simulink subsystem "Simulatorev2slx"  (R2023a)
settings: Solver=VariableStepAuto  StartTime=0.0  StopTime=10.0  RelTol=1e-3
model mask{rho=971, rho_air=971, c_p=4179, c_p_air=4179, pi=3.14151, L_F=40.5, D_F=0.4, h_F=1.5, D_S1=0.1, L_S1=5, h_S1=1.5, D_S2=0.02, L_S2=50, h_S2=1.5, D_S3=0.1, L_S3=5, h_S3=1.5, D_R=0.4, L_R=40, h_R=1.5, V_b=300, A_b=500, h_b=1.5, T_F_0=273, T_S1_0=273, T_S2_0=273, T_S3_0=273, T_b_0=273, T_R_0=273}
  mask prompts: rho "rho water [kg/m^3]"; rho_air "rho air [kg/m^3]"; c_p "c_p water [J/kgK]"; c_p_air "c_p air [J/kgK]"; L_F "Length of F [m]"; D_F "Diameter of F [m]"; h_F "h_F [W/m^2K]"; D_S1 "Diameter of S1 [m]"; L_S1 "Length of S1"; D_S2 "Diameter of S2"; L_S2 "Length of S2"; D_S3 "Diameter of S3"; L_S3 "Length of S3"; D_R "Diameter of R"; L_R "Length of R"; V_b "V_building"; A_b "A_building_hull"; h_b "h_building"
undefined symbols (not defined in the file): C_b, C_F, C_R, C_S1, C_S2, C_S3, k_b, k_F, k_R, k_S1, k_S2, k_S3
settings Model: Creator=alex  LastModifiedBy=alex
settings OptimizationCC: ReuseModelBlockBuffer=off

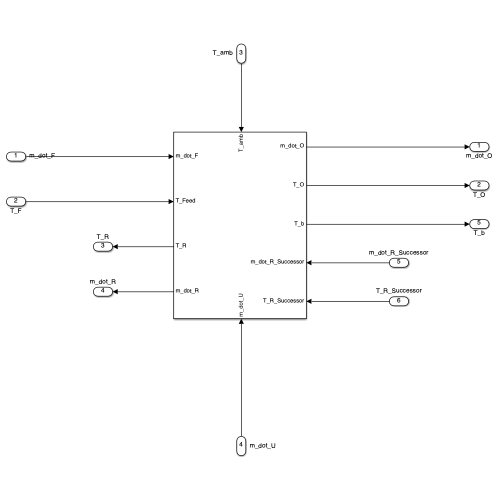
[thumbnail: Simulink's stored preview of the top-level diagram]
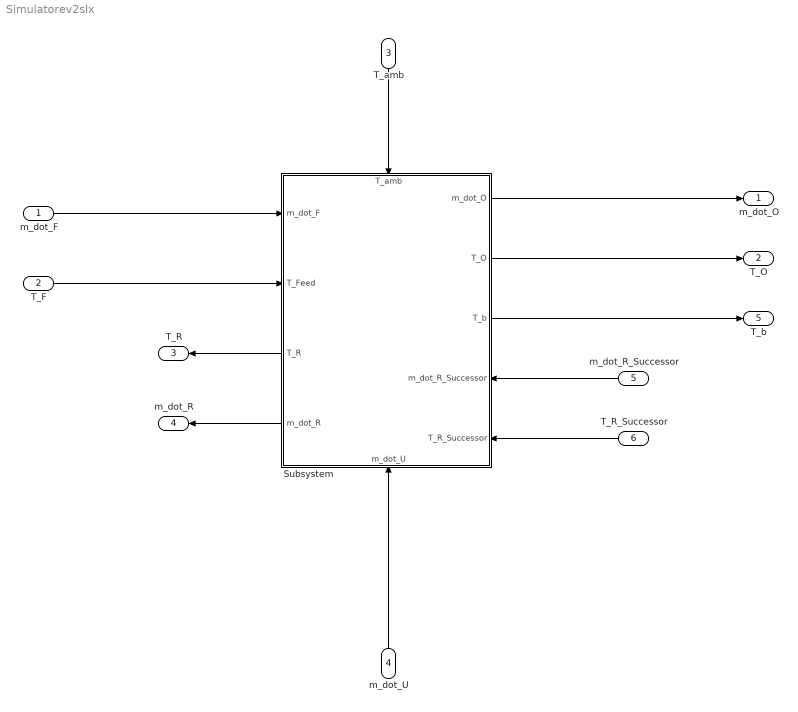
== system Simulatorev2slx ==
  m_dot_F : Inport
  T_F : Inport  Port=2
  T_amb : Inport  Port=3
  m_dot_U : Inport  Port=4
  m_dot_R_Successor : Inport  Port=5
  T_R_Successor : Inport  Port=6
  Subsystem : Subsystem
      settings: PortSchema="{\"entries\":[{\"content\":{\"sides\":[{\"content\":{\"connectorIds\":[\"In1\",\"In2\",\"Out4\",\"Out5\"]},\"type\":\"ConnectorPlacement.EquallySpacedRectSide\",\"uuid\":\"02066a73-e12c-4efb-ac1f-3567aea7908b\"},{\"content\":{\"connectorIds\":[\"Out1\",\"Out2\",\"Out3\",\"In5\",\"In6\"],\"side\":\"RIGHT\"},\"type\":\"ConnectorPlacement.EquallySpacedRectSide\",\"uuid\":\"ccd81727-46b8-449c-bb2a-a5652a5d9084\"},{\"content\":{\"connectorIds\":[\"In3\"],\"side\":\"TOP\"},\"type\":\"ConnectorPlacement.EquallySpacedRectSide\",\"uuid\":\"9b852ef9-fe85-43d4-afda-854933deff9c\"},{\"content\":{\"connectorIds\":[\"In4\"],\"side\":\"BOTTOM\"},\"type\":\"ConnectorPlacement.EquallySpacedRectSide\",\"uuid\":\"c5c6073a-07c2-439b-a52e-85716bb20a3c\"}]},\"type\":\"ConnectorPlacement.EquallySpacedConnector\",\"uuid\":\"28865625-48f4-4f1f-9e76-2e1450716591\"}],\"packageUris\":[\"http://schema.mathworks.com/mf0/Connector/R2020b\"],\"version\":\"1.0\"}"
  m_dot_O : Outport
  T_O : Outport  Port=2
  T_R : Outport  Port=3
  m_dot_R : Outport  Port=4
  T_b : Outport  Port=5
  wires:
  m_dot_F/1 -> Subsystem/1(m_dot_F)
  T_F/1 -> Subsystem/2(T_Feed)
  T_amb/1 -> Subsystem/3(T_amb)
  m_dot_U/1 -> Subsystem/4(m_dot_U)
  Subsystem/1(m_dot_O) -> m_dot_O/1
  Subsystem/2(T_O) -> T_O/1
  m_dot_R_Successor/1 -> Subsystem/5(m_dot_R_Successor)
  T_R_Successor/1 -> Subsystem/6(T_R_Successor)
  Subsystem/4(T_R) -> T_R/1
  Subsystem/5(m_dot_R) -> m_dot_R/1
  Subsystem/3(T_b) -> T_b/1

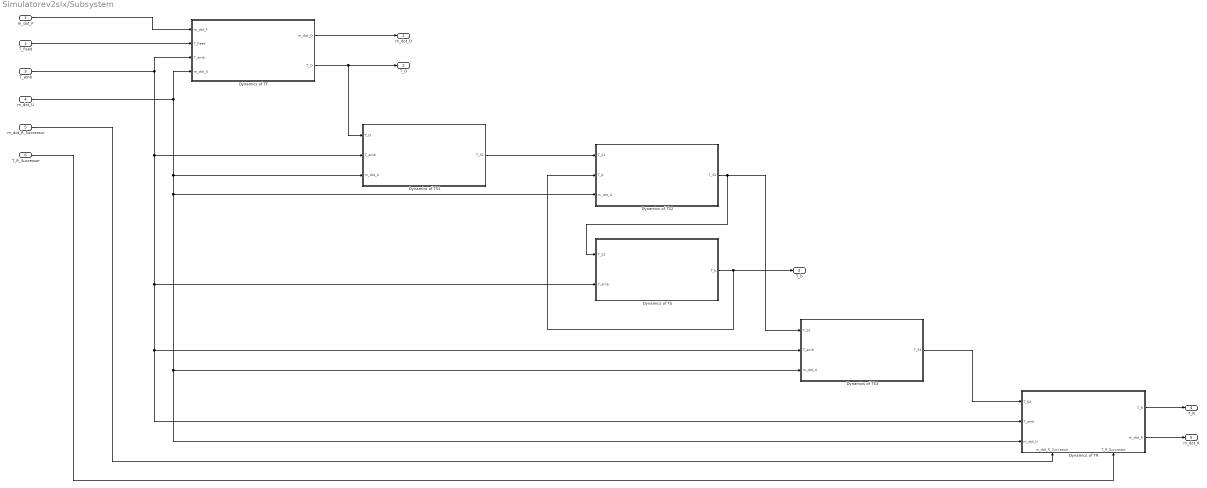
== system Simulatorev2slx/Subsystem ==
  m_dot_F : Inport
  T_Feed : Inport  Port=2
  T_amb : Inport  Port=3
  m_dot_U : Inport  Port=4
  m_dot_R_Successor : Inport  Port=5
  T_R_Successor : Inport  Port=6
  Dynamics of TF : Subsystem
  Dynamics of TR : Subsystem
      settings: PortSchema="{\"entries\":[{\"content\":{\"sides\":[{\"content\":{\"connectorIds\":[\"In1\",\"In2\",\"In3\"]},\"type\":\"ConnectorPlacement.EquallySpacedRectSide\",\"uuid\":\"1d5cfb0c-3444-494a-8f15-ea1ce9aa89e1\"},{\"content\":{\"connectorIds\":[\"Out1\",\"Out2\"],\"side\":\"RIGHT\"},\"type\":\"ConnectorPlacement.EquallySpacedRectSide\",\"uuid\":\"a241c28b-af63-4b6d-8a8e-9e454c2f304f\"},{\"content\":{\"side\":\"TOP\"},\"type\":\"ConnectorPlacement.EquallySpacedRectSide\",\"uuid\":\"7a4239f2-e3be-4ccc-ba79-85038cac89dd\"},{\"content\":{\"connectorIds\":[\"In4\",\"In5\"],\"side\":\"BOTTOM\"},\"type\":\"ConnectorPlacement.EquallySpacedRectSide\",\"uuid\":\"03da5dbc-12e1-4117-b594-812fe8cbcf6d\"}]},\"type\":\"ConnectorPlacement.EquallySpacedConnector\",\"uuid\":\"6bf2d3a5-b163-467e-ac11-ed480dce725b\"}],\"packageUris\":[\"http://schema.mathworks.com/mf0/Connector/R2020b\"],\"version\":\"1.0\"}"
  Dynamics of TS1 : Subsystem
  Dynamics of TS2 : Subsystem
  Dynamics of TS3 : Subsystem
  Dynamics of Tb : Subsystem
  m_dot_O : Outport
  T_O : Outport  Port=2
  T_b : Outport  Port=3
  T_R : Outport  Port=4
  m_dot_R : Outport  Port=5
  wires:
  m_dot_F/1 -> Dynamics of TF/1(m_dot_F)
  T_Feed/1 -> Dynamics of TF/2(T_Feed)
  T_amb/1 -> Dynamics of Tb/2(T_amb), Dynamics of TS3/2(T_amb), Dynamics of TR/2(T_amb), Dynamics of TS1/2(T_amb), Dynamics of TF/3(T_amb)
  m_dot_U/1 -> Dynamics of TR/3(m_dot_U), Dynamics of TS3/3(m_dot_U), Dynamics of TS2/3(m_dot_U), Dynamics of TS1/3(m_dot_U), Dynamics of TF/4(m_dot_U)
  Dynamics of TF/1(m_dot_O) -> m_dot_O/1
  Dynamics of TF/2(T_O) -> Dynamics of TS1/1(T_O), T_O/1
  Dynamics of TS1/1(T_S1) -> Dynamics of TS2/1(T_S1)
  Dynamics of TS2/1(T_S2) -> Dynamics of TS3/1(T_S2), Dynamics of Tb/1(T_S2)
  Dynamics of Tb/1(T_b) -> T_b/1, Dynamics of TS2/2(T_b)
  m_dot_R_Successor/1 -> Dynamics of TR/4(m_dot_R_Successor)
  T_R_Successor/1 -> Dynamics of TR/5(T_R_Successor)
  Dynamics of TS3/1(T_S3) -> Dynamics of TR/1(T_S3)
  Dynamics of TR/1(T_R) -> T_R/1
  Dynamics of TR/2(m_dot_R) -> m_dot_R/1

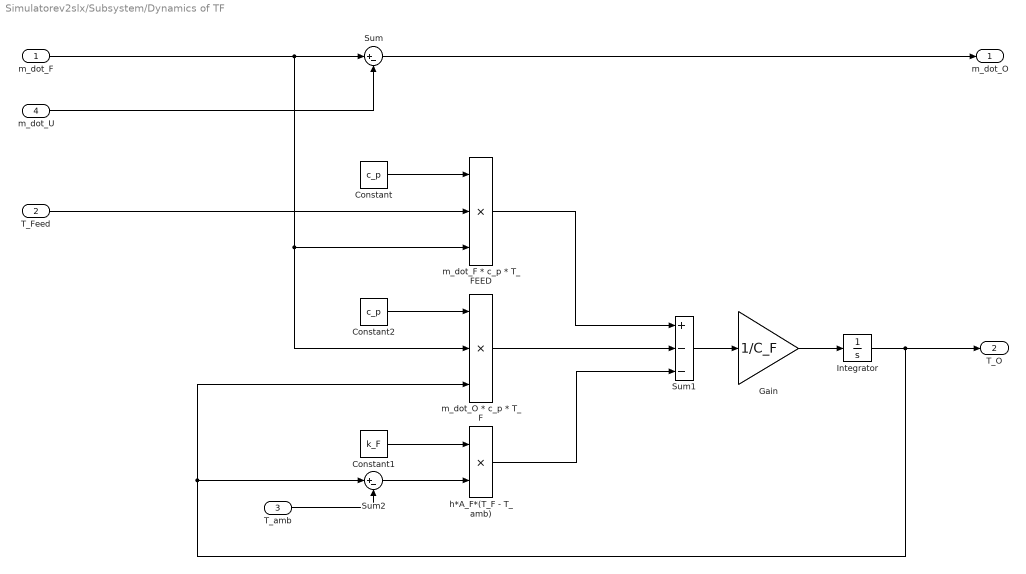
== system Simulatorev2slx/Subsystem/Dynamics of TF ==
  m_dot_F : Inport
  T_Feed : Inport  Port=2
  T_amb : Inport  Port=3
  m_dot_U : Inport  Port=4
  Constant : Constant  Value=c_p
  Constant1 : Constant  Value=k_F
  Constant2 : Constant  Value=c_p
  Gain : Gain  Gain=1/C_F
  Integrator : Integrator  InitialCondition=T_F_0
  Sum : Sum  Inputs=|+-
  Sum1 : Sum  Inputs=+--
  Sum2 : Sum  Inputs=|+-
  h*A_F*(T_F - T_amb) : Product
  m_dot_F * c_p * T_FEED : Product  Inputs=3
  m_dot_O * c_p * T_F : Product  Inputs=3
  m_dot_O : Outport
  T_O : Outport  Port=2
  wires:
  Constant2/1 -> m_dot_O * c_p * T_F/1
  m_dot_O * c_p * T_F/1 -> Sum1/2
  T_amb/1 -> Sum2/2
  Integrator/1 -> T_O/1, m_dot_O * c_p * T_F/3, Sum2/1
  Constant1/1 -> h*A_F*(T_F - T_amb)/1
  h*A_F*(T_F - T_amb)/1 -> Sum1/3
  Sum2/1 -> h*A_F*(T_F - T_amb)/2
  m_dot_F * c_p * T_FEED/1 -> Sum1/1
  Constant/1 -> m_dot_F * c_p * T_FEED/1
  Sum1/1 -> Gain/1
  m_dot_F/1 -> m_dot_F * c_p * T_FEED/3, m_dot_O * c_p * T_F/2, Sum/1
  Gain/1 -> Integrator/1
  Sum/1 -> m_dot_O/1
  T_Feed/1 -> m_dot_F * c_p * T_FEED/2
  m_dot_U/1 -> Sum/2

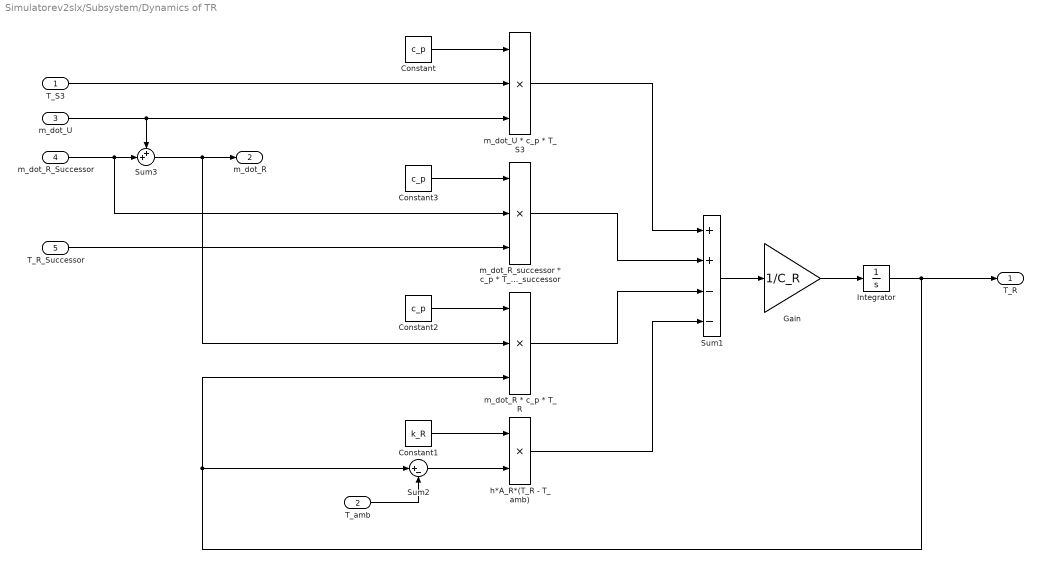
== system Simulatorev2slx/Subsystem/Dynamics of TR ==
  T_S3 : Inport
  T_amb : Inport  Port=2
  m_dot_U : Inport  Port=3
  m_dot_R_Successor : Inport  Port=4
  T_R_Successor : Inport  Port=5
  Constant : Constant  Value=c_p
  Constant1 : Constant  Value=k_R
  Constant2 : Constant  Value=c_p
  Constant3 : Constant  Value=c_p
  Gain : Gain  Gain=1/C_R
  Integrator : Integrator  InitialCondition=T_R_0
  Sum1 : Sum  Inputs=++--
  Sum2 : Sum  Inputs=|+-
  Sum3 : Sum  Inputs=++|
  h*A_R*(T_R - T_amb) : Product
  m_dot_R * c_p * T_R : Product  Inputs=3
  m_dot_R_successor * c_p * T_R_successor : Product  Inputs=3
  m_dot_U * c_p * T_S3 : Product  Inputs=3
  T_R : Outport
  m_dot_R : Outport  Port=2
  wires:
  Constant2/1 -> m_dot_R * c_p * T_R/1
  T_amb/1 -> Sum2/2
  Integrator/1 -> T_R/1, m_dot_R * c_p * T_R/3, Sum2/1
  Constant1/1 -> h*A_R*(T_R - T_amb)/1
  Sum2/1 -> h*A_R*(T_R - T_amb)/2
  Constant/1 -> m_dot_U * c_p * T_S3/1
  Sum1/1 -> Gain/1
  Gain/1 -> Integrator/1
  T_S3/1 -> m_dot_U * c_p * T_S3/2
  m_dot_U/1 -> m_dot_U * c_p * T_S3/3, Sum3/1
  Sum3/1 -> m_dot_R * c_p * T_R/2, m_dot_R/1
  m_dot_R_Successor/1 -> m_dot_R_successor * c_p * T_R_successor/2, Sum3/2
  Constant3/1 -> m_dot_R_successor * c_p * T_R_successor/1
  T_R_Successor/1 -> m_dot_R_successor * c_p * T_R_successor/3
  h*A_R*(T_R - T_amb)/1 -> Sum1/4
  m_dot_R * c_p * T_R/1 -> Sum1/3
  m_dot_R_successor * c_p * T_R_successor/1 -> Sum1/2
  m_dot_U * c_p * T_S3/1 -> Sum1/1

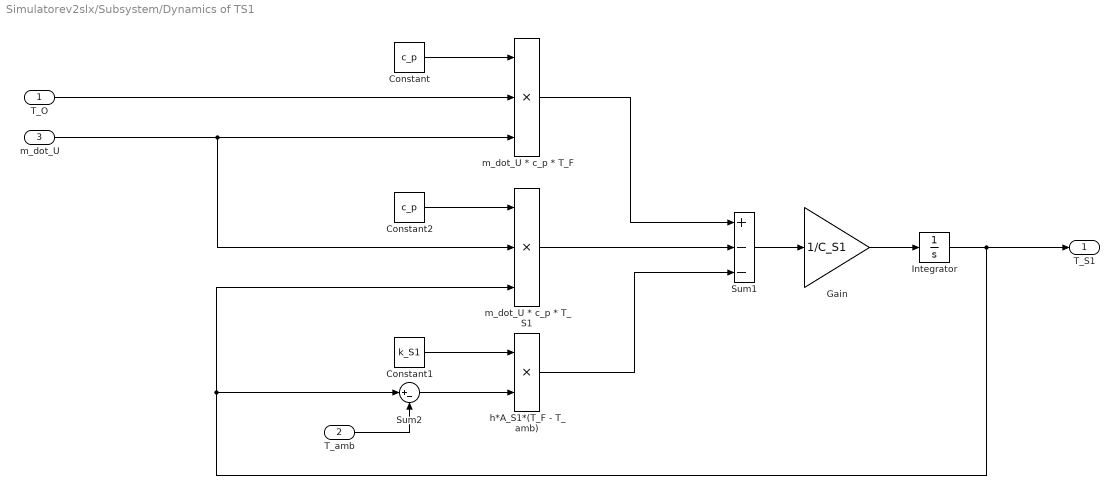
== system Simulatorev2slx/Subsystem/Dynamics of TS1 ==
  T_O : Inport
  T_amb : Inport  Port=2
  m_dot_U : Inport  Port=3
  Constant : Constant  Value=c_p
  Constant1 : Constant  Value=k_S1
  Constant2 : Constant  Value=c_p
  Gain : Gain  Gain=1/C_S1
  Integrator : Integrator  InitialCondition=T_S1_0
  Sum1 : Sum  Inputs=+--
  Sum2 : Sum  Inputs=|+-
  h*A_S1*(T_F - T_amb) : Product
  m_dot_U * c_p * T_F : Product  Inputs=3
  m_dot_U * c_p * T_S1 : Product  Inputs=3
  T_S1 : Outport
  wires:
  Constant2/1 -> m_dot_U * c_p * T_S1/1
  m_dot_U * c_p * T_S1/1 -> Sum1/2
  T_amb/1 -> Sum2/2
  Integrator/1 -> T_S1/1, m_dot_U * c_p * T_S1/3, Sum2/1
  Constant1/1 -> h*A_S1*(T_F - T_amb)/1
  h*A_S1*(T_F - T_amb)/1 -> Sum1/3
  Sum2/1 -> h*A_S1*(T_F - T_amb)/2
  m_dot_U * c_p * T_F/1 -> Sum1/1
  Constant/1 -> m_dot_U * c_p * T_F/1
  Sum1/1 -> Gain/1
  Gain/1 -> Integrator/1
  T_O/1 -> m_dot_U * c_p * T_F/2
  m_dot_U/1 -> m_dot_U * c_p * T_S1/2, m_dot_U * c_p * T_F/3

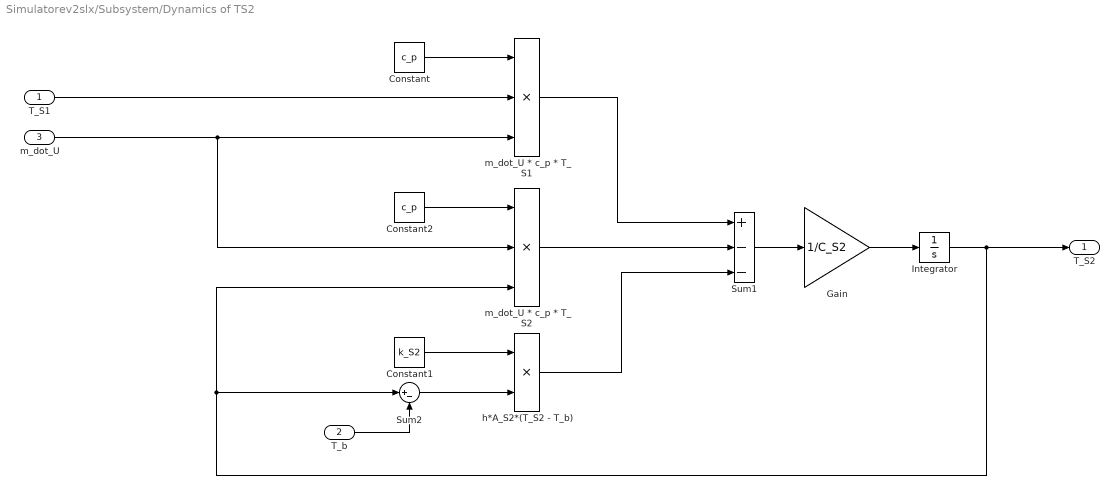
== system Simulatorev2slx/Subsystem/Dynamics of TS2 ==
  T_S1 : Inport
  T_b : Inport  Port=2
  m_dot_U : Inport  Port=3
  Constant : Constant  Value=c_p
  Constant1 : Constant  Value=k_S2
  Constant2 : Constant  Value=c_p
  Gain : Gain  Gain=1/C_S2
  Integrator : Integrator  InitialCondition=T_S2_0
  Sum1 : Sum  Inputs=+--
  Sum2 : Sum  Inputs=|+-
  h*A_S2*(T_S2 - T_b) : Product
  m_dot_U * c_p * T_S1 : Product  Inputs=3
  m_dot_U * c_p * T_S2 : Product  Inputs=3
  T_S2 : Outport
  wires:
  Constant2/1 -> m_dot_U * c_p * T_S2/1
  m_dot_U * c_p * T_S2/1 -> Sum1/2
  T_b/1 -> Sum2/2
  Integrator/1 -> T_S2/1, m_dot_U * c_p * T_S2/3, Sum2/1
  Constant1/1 -> h*A_S2*(T_S2 - T_b)/1
  h*A_S2*(T_S2 - T_b)/1 -> Sum1/3
  Sum2/1 -> h*A_S2*(T_S2 - T_b)/2
  m_dot_U * c_p * T_S1/1 -> Sum1/1
  Constant/1 -> m_dot_U * c_p * T_S1/1
  Sum1/1 -> Gain/1
  Gain/1 -> Integrator/1
  T_S1/1 -> m_dot_U * c_p * T_S1/2
  m_dot_U/1 -> m_dot_U * c_p * T_S2/2, m_dot_U * c_p * T_S1/3

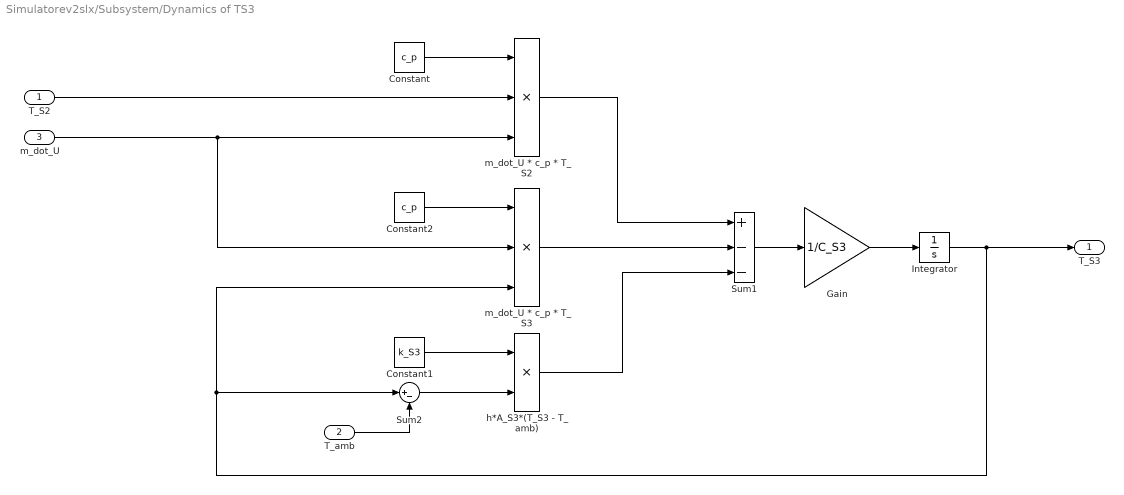
== system Simulatorev2slx/Subsystem/Dynamics of TS3 ==
  T_S2 : Inport
  T_amb : Inport  Port=2
  m_dot_U : Inport  Port=3
  Constant : Constant  Value=c_p
  Constant1 : Constant  Value=k_S3
  Constant2 : Constant  Value=c_p
  Gain : Gain  Gain=1/C_S3
  Integrator : Integrator  InitialCondition=T_S3_0
  Sum1 : Sum  Inputs=+--
  Sum2 : Sum  Inputs=|+-
  h*A_S3*(T_S3 - T_amb) : Product
  m_dot_U * c_p * T_S2 : Product  Inputs=3
  m_dot_U * c_p * T_S3 : Product  Inputs=3
  T_S3 : Outport
  wires:
  Constant2/1 -> m_dot_U * c_p * T_S3/1
  m_dot_U * c_p * T_S3/1 -> Sum1/2
  T_amb/1 -> Sum2/2
  Integrator/1 -> T_S3/1, m_dot_U * c_p * T_S3/3, Sum2/1
  Constant1/1 -> h*A_S3*(T_S3 - T_amb)/1
  h*A_S3*(T_S3 - T_amb)/1 -> Sum1/3
  Sum2/1 -> h*A_S3*(T_S3 - T_amb)/2
  m_dot_U * c_p * T_S2/1 -> Sum1/1
  Constant/1 -> m_dot_U * c_p * T_S2/1
  Sum1/1 -> Gain/1
  Gain/1 -> Integrator/1
  T_S2/1 -> m_dot_U * c_p * T_S2/2
  m_dot_U/1 -> m_dot_U * c_p * T_S3/2, m_dot_U * c_p * T_S2/3

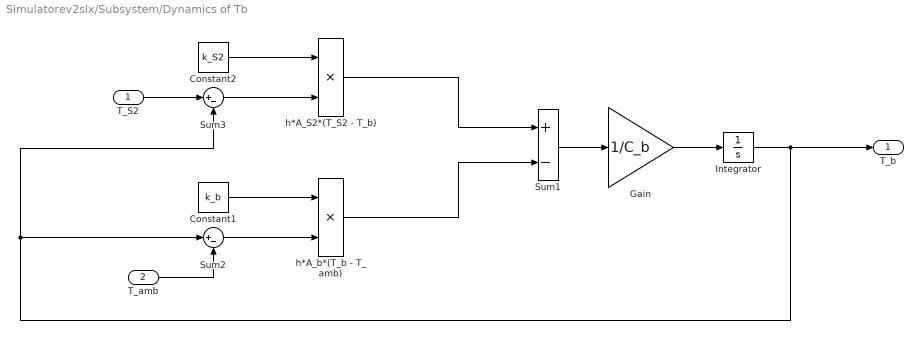
== system Simulatorev2slx/Subsystem/Dynamics of Tb ==
  T_S2 : Inport
  T_amb : Inport  Port=2
  Constant1 : Constant  Value=k_b
  Constant2 : Constant  Value=k_S2
  Gain : Gain  Gain=1/C_b
  Integrator : Integrator  InitialCondition=T_b_0
  Sum1 : Sum  Inputs=+-
  Sum2 : Sum  Inputs=|+-
  Sum3 : Sum  Inputs=|+-
  h*A_S2*(T_S2 - T_b) : Product
  h*A_b*(T_b - T_amb) : Product
  T_b : Outport
  wires:
  T_amb/1 -> Sum2/2
  Integrator/1 -> T_b/1, Sum3/2, Sum2/1
  Constant1/1 -> h*A_b*(T_b - T_amb)/1
  Sum2/1 -> h*A_b*(T_b - T_amb)/2
  Sum1/1 -> Gain/1
  Gain/1 -> Integrator/1
  Sum3/1 -> h*A_S2*(T_S2 - T_b)/2
  Constant2/1 -> h*A_S2*(T_S2 - T_b)/1
  h*A_b*(T_b - T_amb)/1 -> Sum1/2
  T_S2/1 -> Sum3/1
  h*A_S2*(T_S2 - T_b)/1 -> Sum1/1
